simulink model "CM640A_MotAg1Meas"  (R2013b)
settings: Solver=FixedStepDiscrete  SolverMode=SingleTasking  StartTime=0.0  StopTime=1  FixedStep=0.0000625  RelTol=1e-3
undefined symbols (not defined in the file): ARCHGLBPRM_2PI_ULS_F32, COEFFTBLELMSIZE_CNT_U08, COEFFTBLSIZE_CNT_U08, CORRNTBLAGSTEPSIZE_MATRAD_F32, CORRNTBLSIDXOFFS_CNT_U16, CORRNTBLSIZE_CNT_U16, CORRNTBLSIZEMASK_CNT_U08, MOTAG1OFFS_MOTREV_U0P16, MotAg1PrtclFlt, MOTAG1PRTCLFLTFAILSTEP_CNT_U16, MOTAG1PRTCLFLTPASSSTEP_CNT_U16, MOTAGDELTAPERCORRNPT_CNT_U16, MOTAGIDXMASK_CNT_U16, MotCtrlMotAg1ErrReg, NtcSts1, sigbuilder_block, SNSRAGMASK_CNT_U32, SNSRERRMASK_CNT_U32, SNSRERRNTCMASK_CNT_U08, SNSRVLTGFLTMASK_CNT_U32, SPIPARMASK_CNT_U32
libraries: simulink x28, FloatToFixd x1, NxtrMax x1, NxtrLim x1
(part 1 of 4)
settings Model: RequirementInfo="{}  %GIDa_ca294f38_ed7c_4fb9_8c54_f4d56271bfc7"  ModifiedHistory=Rev 008: Updated model to Matlab 2013B, added comments to show requirement linkage  Creator=nz3zln  LastModifiedBy=FZG88Y
settings SolverCC: AutoInsertRateTranBlk=on  InsertRTBMode=Always
settings DataIOCC: LimitDataPoints=off  SaveFormat=Structure  ReturnWorkspaceOutputs=on
settings OptimizationCC: BlockReduction=off  InlineParams=on  ZeroExternalMemoryAtStartup=off  ZeroInternalMemoryAtStartup=off  OptimizeModelRefInitCode=on  LifeSpan=1
settings DebuggingCC: SignalInfNanChecking=error  SignalRangeChecking=warning  UnderspecifiedInitializationDetection=Simplified  SolverPrmCheckMsg=error  InheritedTsInSrcMsg=error  DiscreteInheritContinuousMsg=error  SingleTaskRateTransMsg=error  TasksWithSamePriorityMsg=error  SigSpecEnsureSampleTimeMsg=error  CheckMatrixSingularityMsg=error  ParameterUnderflowMsg=error  ParameterPrecisionLossMsg=error  ParameterTunabilityLossMsg=error  FixptConstUnderflowMsg=warning  FixptConstOverflowMsg=warning  VectorMatrixConversionMsg=error  SignalLabelMismatchMsg=error  UnconnectedInputMsg=error  UnconnectedOutputMsg=error  UnconnectedLineMsg=error  SFcnCompatibilityMsg=error  UniqueDataStoreMsg=warning  BusObjectLabelMismatch=error  RootOutportRequireBusObject=error  AssertControl=DisableAll  ModelReferenceIOMsg=error  ModelReferenceVersionMismatchMessage=warning  ModelReferenceIOMismatchMessage=error  ModelReferenceCSMismatchMessage=warning  ModelReferenceDataLoggingMessage=error  StateNameClashWarn=warning  StrictBusMsg=ErrorOnBusTreatedAsVector  NonBusSignalsTreatedAsBus=error  SFUnexpectedBacktrackingDiag=error  SFInvalidInputDataAccessInChartInitDiag=error  SFNoUnconditionalDefaultTransitionDiag=error  SFTransitionOutsideNaturalParentDiag=error  SFUnconditionalTransitionShadowingDiag=error  SFUndirectedBroadcastEventsDiag=error
settings ModelReferenceCC: ModelReferenceNumInstancesAllowed=Single
settings RTWCC: SystemTargetFile=autosar.tlc  GenCodeOnly=on  TemplateMakefile=ert_default_tmf  Description=AUTOSAR  GenerateReport=on  ProcessScript=autosar_make_rtw_hook  LaunchReport=on
settings CodeAppCC: GenerateComments=off  IgnoreCustomStorageClasses=off  CustomSymbolStrType=$N$R$M  CustomSymbolStrBlkIO=$N$M  SimulinkBlockComments=off
settings STFCustomTargetCC: ParMdlRefBuildCompliant=on  CompOptLevelCompliant=on  IncludeMdlTerminateFcn=off  CombineOutputUpdateFcns=on  SuppressErrorStatus=on  ERTFirstTimeCompliant=on  ERTCustomFileBanners=on  SupportNonFinite=off  SupportComplex=off  SupportContinuousTime=off  SupportNonInlinedSFcns=off  MATLABClassNameForMDSCustomization=Simulink.SoftwareTarget.ERTCustomization  AutosarCompliant=on  GRTInterface=off  SystemTargetFile=autosar.tlc
settings ERTTargetCC: CodeReplacementLibrary=ANSI_C  ConcurrentExecutionCompliant=off  IncludeMdlTerminateFcn=off  SuppressErrorStatus=on  SupportNonFinite=off  SupportComplex=off  ModelStepFunctionPrototypeControlCompliant=off  CPPClassGenCompliant=off  AutosarCompliant=on  InlinedParameterPlacement=NonHierarchical  ERTCustomFileTemplate=example_file_process.tlc  EnableUserReplacementTypes=on

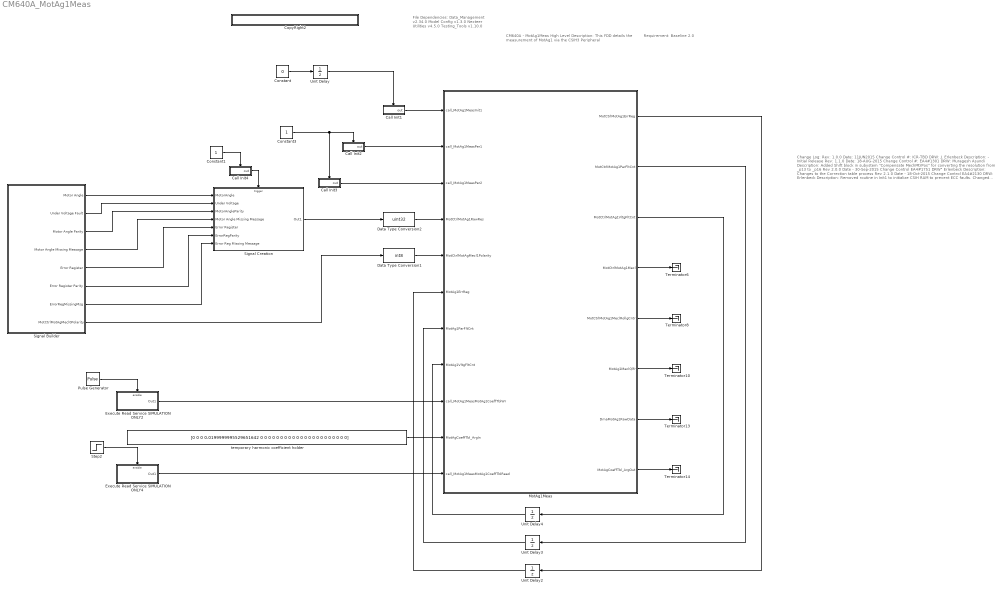
== system CM640A_MotAg1Meas ==
  note: CM640A - MotAg1Meas
      |
      | High Level Description:
      | This FDD details the measurement of MotAg1 via the CSIH3 Peripheral
  note: Change Log:
      |
      | Rev: 1.0.0
      | Date: 11JUN2015
      | Change Control #: ICR-TBD
      | DRW: J. Erlenbeck
      | Description:
      | - Initial Release
      |
      | Rev: 1.1.0
      | Date: 18-AUG-2015
      | Change Control #: EA4#1301
      | DRW: Muragesh Asundi
      | Description: Added Shift block in subystem "Compensate MechMtrPos" for converting the resolution from _p13 to _p16
      |
      | Rev 2.0.0
      | Date - 30-Sep-2015
      | Change Control EA4#1751
      | DRW" Erlenbeck
      | Description: Changes to the Correction table process
      |
      | Rev 2.1.0
      | Date -  18-Oct-2015
      | Change Control EA4#2130
      | DRW: Erlenbeck
      | Description: Removed routine in Init1 to initialize CSIH RAM to prevent ECC faults.  Changed some
      | typecasting in init function that prevented the function from running when NxtrMBDConfig.mat was run.
      | Replaced input signal creation from external file to one with signal builder.
      |
      | Rev 2.4.0
      | Date -  17-Dec-2015
      | Change Control EA4#3209
      | DRW: Erlenbeck
      | Description: Removed read reset pointer
      |
      | Rev 2.5.0
      | Date -  08-Mar-2016
      | Change Control EA4#3999, EA4#4646
      | DRW: Praveen(KPIT)
      | Description: -
      | - M File change so that NVM MotAg1CoeffTbl.EngInit = []. Accordingly model updated to allign to this.
      | - As per anomaly CR EA4#3631, updated the Variable MotCtrlMotAg1VltgFltCnt.WrittenIn field as MotAg1MeasPer1 in the .m file.
      | - The maximum and minimum specified in the Data Type conversion block are removed and highlighted in the Model.
      | - Server runnable name changed from MotAg0MeasMotAg1CoeffTblRead to MotAg1MeasMotAg1CoeffTblRead.
  note: File Dependencies:
      | Data_Management v2.34.0
      | Model Config v1.3.0
      | Nexteer Utilities v4.5.0
      | Testing_Tools v1.10.0
  note: Requirement: Baseline 2.0
  Call Init1 : Subsystem  TreatAsAtomicUnit=on
  Call Init2 : Subsystem  TreatAsAtomicUnit=on
  Call Init3 : Subsystem  TreatAsAtomicUnit=on
  Call Init4 : Subsystem  TreatAsAtomicUnit=on
  Constant : Constant  Value=0  OutDataTypeStr=uint8
  Constant1 : Constant  OutDataTypeStr=int8
  Constant3 : Constant  OutDataTypeStr=int8
  CopyRight2 : Subsystem  Description=|  mask(Copyright Information){none=on}
      | Copyright info block.                                               
      |                                                                     
      | Place copyright information at the top of every subsystem in design.
      mask prompts: none "No parameters"
      mask help: Place copyright information at the top of every subsystem in design.
      mask Display:
      | NxtrConf = 'Nexteer Confidential';
      | 
      | sys = bdroot; %handle for the current model ("system")
      | first = get_param(sys,'Created');
      | first = first(end-3:end);  %year is last four digits
      | 
      | last = get_param(sys,'LastModifiedDate');
      | if isempty(last)
      |     last = datestr(now,'yyyy');
      | else
      |     last = last(end-3:end);
      | end
      | 
      | if strcmp(first,last)
      |     fprintf('%s -- Copyright %s Nexteer',NxtrConf,first)
      | else
      |     fprintf('%s -- %s%s- %s Nexteer',NxtrConf,char(169),first,last)
      | end
  Data Type Conversion1 : DataTypeConversion  OutDataTypeStr=int8
  Data Type Conversion2 : DataTypeConversion  OutDataTypeStr=uint32
  Execute Read Service SIMULATION ONLY2 : Subsystem  TreatAsAtomicUnit=on
  Execute Read Service SIMULATION ONLY4 : Subsystem  TreatAsAtomicUnit=on
  MotAg1Meas : Subsystem
  Pulse Generator : DiscretePulseGenerator  PulseType=Time based  Period=1  PhaseDelay=0.6
  Signal Builder : Subsystem  Tag=STV Subsys  LoadFcn=sigbuilder_block('load');  StartFcn=sigbuilder_block('start');  StopFcn=sigbuilder_block('stop');  ClipboardFcn=sigbuilder_block('clipboard');  mask(Sigbuilder block){}
      mask help: Simulink:masks:SigbuilderBlock_MD
      mask init:
      | if ~strcmp(get_param(bdroot(gcbh),'SimulationStatus'),'stopped') tuvar = sigbuilder_block('maskInit'); end
      settings: CopyFcn=sigbuilder_block('copy');  DeleteFcn=sigbuilder_block('delete');  ModelCloseFcn=sigbuilder_block('modelClose');  PreSaveFcn=sigbuilder_block('preSave');  PauseFcn=sigbuilder_block('pause');  ContinueFcn=sigbuilder_block('continue');  NameChangeFcn=sigbuilder_block('namechange');  OpenFcn=sigbuilder_block('open',[306 215.379 548.69 396.621 ]);  CloseFcn=sigbuilder_block('close');
      mask Display: plot(0, 0, 100, 100,[2, 2, 32, 32, 2], [68, 8, 8, 68, 68],[32, 2], [38, 38], [32, 19, 2],[53, 60, 44], [32, 17, 17, 2],[16, 16, 31, 31]);txt = getActiveGroup(gcbh);text(2, 100, txt,'verticalAlignment', 'top');
  Signal Creation : Subsystem
  Step2 : Step  Time=0.8  SampleTime=0
  Terminator{6,8,10,13..14} (5 alike) : Terminator
  Unit Delay : UnitDelay  InitialCondition=1  SampleTime=-1
  Unit Delay2 : UnitDelay  SampleTime=-1
  Unit Delay3 : UnitDelay  SampleTime=-1
  Unit Delay4 : UnitDelay  SampleTime=-1
  temporary harmonic coefficient holder : Constant  Value=[0 0 0 0.0199999995529651642 0 0 0 0 0 0 0 0 0 0 0 0 0 0 0 0 0 0 0 0 0 0]  OutDataTypeStr=single
  wires:
  Constant/1 -> Unit Delay/1
  Unit Delay/1 -> Call Init1/Enable
  Constant3/1 -> Call Init2/Enable, Call Init3/Enable
  Call Init1/1(out) -> MotAg1Meas/1(call_MotAg1MeasInit1)
  Call Init2/1(out) -> MotAg1Meas/2(call_MotAg1MeasPer1)
  Call Init3/1(out) -> MotAg1Meas/3(call_MotAg1MeasPer2)
  MotAg1Meas/4(MotCtrlMotAg1Mecl) -> Terminator6/1
  MotAg1Meas/5(MotCtrlMotAg1MeclRollgCntr) -> Terminator8/1
  MotAg1Meas/6(MotAg1MeclQlfr) -> Terminator10/1
  MotAg1Meas/7(DmaMotAg1RawData) -> Terminator13/1
  Pulse Generator/1 -> Execute Read Service SIMULATION ONLY2/Enable
  Step2/1 -> Execute Read Service SIMULATION ONLY4/Enable
  MotAg1Meas/1(MotCtrlMotAg1ErrReg) -> Unit Delay2/1
  Unit Delay2/1 -> MotAg1Meas/6(MotAg1ErrReg)
  MotAg1Meas/2(MotCtrlMotAg1ParFltCnt) -> Unit Delay3/1
  Unit Delay3/1 -> MotAg1Meas/7(MotAg1ParFltCnt)
  MotAg1Meas/3(MotCtrlMotAg1VltgFltCnt) -> Unit Delay4/1
  Unit Delay4/1 -> MotAg1Meas/8(MotAg1VltgFltCnt)
  MotAg1Meas/8(MotAgCoeffTbl_ArgOut) -> Terminator14/1
  Execute Read Service SIMULATION ONLY2/1(Out1) -> MotAg1Meas/9(call_MotAg1MeasMotAg1CoeffTblWr)
  Execute Read Service SIMULATION ONLY4/1(Out1) -> MotAg1Meas/11(call_MotAg1MeasMotAg1CoeffTblRead)
  temporary harmonic coefficient holder/1 -> MotAg1Meas/10(MotAgCoeffTbl_ArgIn)
  Signal Creation/1(Out1) -> Data Type Conversion2/1
  Constant1/1 -> Call Init4/Enable
  Call Init4/1(out) -> Signal Creation/Trigger
  Signal Builder/1(Motor Angle) -> Signal Creation/1(MotorAngle)
  Signal Builder/2(Under Voltage Fault) -> Signal Creation/2(Under Voltage)
  Signal Builder/3(Motor Angle Parity) -> Signal Creation/3(MotorAngleParity)
  Signal Builder/5(Error Register) -> Signal Creation/5(Error Register)
  Signal Builder/6(Error Register Parity) -> Signal Creation/6(ErrorRegParity)
  Signal Builder/8(MotCtrlMotAgMecl0Polarity) -> Data Type Conversion1/1
  Signal Builder/4(Motor Angle Missing Message) -> Signal Creation/4(Motor Angle Missing Message)
  Signal Builder/7(ErrorRegMissingMsg) -> Signal Creation/7(Error Reg Missing Message)
  Data Type Conversion2/1 -> MotAg1Meas/4(MotCtrlMotAg1RawRes)
  Data Type Conversion1/1 -> MotAg1Meas/5(MotCtrlMotAgMecl1Polarity)

== system CM640A_MotAg1Meas/Call Init1 ==
  Enable : EnablePort
  Function Call Trigger : simulink/Ports & Subsystems/Function-Call Generator  RequirementInfo={} %GIDa_ff755a2e_49d1_45f7_8591_3ce0ef475338  sample_time=0.002  numberOfIterations=1
  out : Outport
  wires:
  Function Call Trigger/1 -> out/1

== system CM640A_MotAg1Meas/Call Init2 ==
  Enable : EnablePort
  Function Call Trigger : simulink/Ports & Subsystems/Function-Call Generator  RequirementInfo={} %GIDa_6dd05ab1_f91b_4d7a_a0ec_1170d213fa7b  sample_time=0.0005  numberOfIterations=1
  out : Outport
  wires:
  Function Call Trigger/1 -> out/1

== system CM640A_MotAg1Meas/Call Init3 ==
  Enable : EnablePort
  Function Call Trigger : simulink/Ports & Subsystems/Function-Call Generator  RequirementInfo={} %GIDa_9bd65ccd_39f3_4e48_9d09_4984d13bbcbb  sample_time=0.002  numberOfIterations=1
  out : Outport
  wires:
  Function Call Trigger/1 -> out/1

== system CM640A_MotAg1Meas/Call Init4 ==
  Enable : EnablePort
  Function Call Trigger : simulink/Ports & Subsystems/Function-Call Generator  RequirementInfo={} %GIDa_6dd05ab1_f91b_4d7a_a0ec_1170d213fa7b  sample_time=0.0005  numberOfIterations=1
  out : Outport
  wires:
  Function Call Trigger/1 -> out/1

== system CM640A_MotAg1Meas/CopyRight2 ==

== system CM640A_MotAg1Meas/Execute Read Service SIMULATION ONLY2 ==
  Enable : EnablePort
  Function-Call Generator1 : simulink/Ports & Subsystems/Function-Call Generator  sample_time=0.0000625  numberOfIterations=1
  Out1 : Outport
  wires:
  Function-Call Generator1/1 -> Out1/1

== system CM640A_MotAg1Meas/Execute Read Service SIMULATION ONLY4 ==
  Enable : EnablePort
  Function-Call Generator1 : simulink/Ports & Subsystems/Function-Call Generator  sample_time=0.0000625  numberOfIterations=1
  Out1 : Outport
  wires:
  Function-Call Generator1/1 -> Out1/1

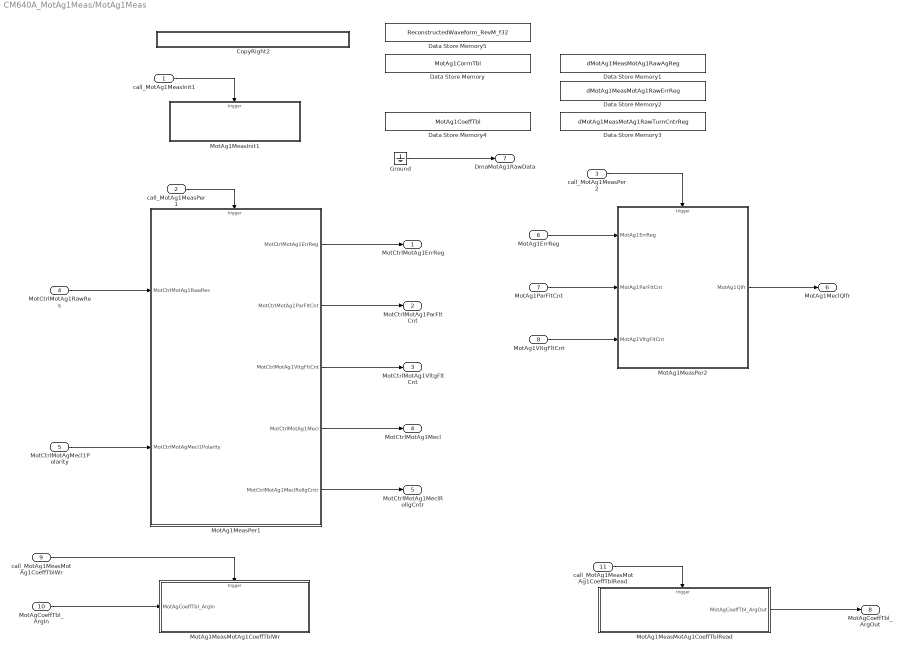
== system CM640A_MotAg1Meas/MotAg1Meas ==
  call_MotAg1MeasInit1 : Inport  RequirementInfo={} %GIDa_18b4b7a7_d8ff_42fd_afd9_8fbc558fb7ae
  call_MotAg1MeasPer1 : Inport  RequirementInfo={} %GIDa_8c56c68f_1996_47ee_bda4_35b4dc112bcf  Port=2
  call_MotAg1MeasPer2 : Inport  RequirementInfo={} %GIDa_7b28921c_189e_46dc_b03b_f7509365a7f9  Port=3
  MotCtrlMotAg1RawRes : Inport  RequirementInfo={} %GIDa_768985a4_e900_425c_ae1d_47338650e664  Port=4
  MotCtrlMotAgMecl1Polarity : Inport  RequirementInfo={} %GIDa_8ed9d5d5_f39e_4ce8_8e17_7324d3fb8e4d  Port=5  OutDataTypeStr=int8
  MotAg1ErrReg : Inport  Port=6
  MotAg1ParFltCnt : Inport  Port=7
  MotAg1VltgFltCnt : Inport  Port=8
  call_MotAg1MeasMotAg1CoeffTblWr : Inport  Port=9
  MotAgCoeffTbl_ArgIn : Inport  Port=10
  call_MotAg1MeasMotAg1CoeffTblRead : Inport  Port=11
  CopyRight2 : Subsystem  Description=|  mask(Copyright Information){none=on}
      | Copyright info block.                                               
      |                                                                     
      | Place copyright information at the top of every subsystem in design.
      mask prompts: none "No parameters"
      mask help: Place copyright information at the top of every subsystem in design.
      mask Display:
      | NxtrConf = 'Nexteer Confidential';
      | 
      | sys = bdroot; %handle for the current model ("system")
      | first = get_param(sys,'Created');
      | first = first(end-3:end);  %year is last four digits
      | 
      | last = get_param(sys,'LastModifiedDate');
      | if isempty(last)
      |     last = datestr(now,'yyyy');
      | else
      |     last = last(end-3:end);
      | end
      | 
      | if strcmp(first,last)
      |     fprintf('%s -- Copyright %s Nexteer',NxtrConf,first)
      | else
      |     fprintf('%s -- %s%s- %s Nexteer',NxtrConf,char(169),first,last)
      | end
  Data Store Memory : DataStoreMemory  DataStoreName=MotAg1CorrnTbl  InitialValue=[]  StateMustResolveToSignalObject=on
  Data Store Memory1 : DataStoreMemory  DataStoreName=dMotAg1MeasMotAg1RawAgReg  OutDataTypeStr=uint32  StateMustResolveToSignalObject=on
  Data Store Memory2 : DataStoreMemory  DataStoreName=dMotAg1MeasMotAg1RawErrReg  OutDataTypeStr=uint32  StateMustResolveToSignalObject=on
  Data Store Memory3 : DataStoreMemory  DataStoreName=dMotAg1MeasMotAg1RawTurnCntrReg  OutDataTypeStr=uint32  StateMustResolveToSignalObject=on
  Data Store Memory4 : DataStoreMemory  DataStoreName=MotAg1CoeffTbl  InitialValue=[]  StateMustResolveToSignalObject=on
  Data Store Memory5 : DataStoreMemory  DataStoreName=ReconstructedWaveform_RevM_f32  InitialValue=zeros(128,1)  OutDataTypeStr=single
  Ground : Ground
  MotAg1MeasInit1 : Subsystem
  MotAg1MeasMotAg1CoeffTblRead : Subsystem  RequirementInfo="{'linktype_rmi_doors' '0000cf48 (/ESG Group/FDD Module Requirements/EA4 Specific/CM640A_MotAg1Meas)' '#CM640A_116' 'true' 'REQ:  CM640A_116' '' } %GIDa_cbbcdd8d_f009_454c_a06b_3b2ba8e819d4"
  MotAg1MeasMotAg1CoeffTblWr : Subsystem  RequirementInfo="{'linktype_rmi_doors' '0000cf48 (/ESG Group/FDD Module Requirements/EA4 Specific/CM640A_MotAg1Meas)' '#CM640A_115' 'true' 'REQ:  CM640A_115' '' } %GIDa_0a2db888_59fe_4955_b15e_b7f61818f82e"
  MotAg1MeasPer1 : Subsystem  TreatAsAtomicUnit=on
  MotAg1MeasPer2 : Subsystem  TreatAsAtomicUnit=on
  MotCtrlMotAg1ErrReg : Outport
  MotCtrlMotAg1ParFltCnt : Outport  Port=2
  MotCtrlMotAg1VltgFltCnt : Outport  Port=3
  MotCtrlMotAg1Mecl : Outport  RequirementInfo={} %GIDa_a40ef296_4e6e_4397_997e_05fcb9e70ed5  Port=4
  MotCtrlMotAg1MeclRollgCntr : Outport  Port=5
  MotAg1MeclQlfr : Outport  RequirementInfo={} %GIDa_eb095ceb_60c6_4658_947c_a9047682a36a  Port=6
  DmaMotAg1RawData : Outport  Port=7
  MotAgCoeffTbl_ArgOut : Outport  Port=8
  wires:
  MotCtrlMotAgMecl1Polarity/1 -> MotAg1MeasPer1/2(MotCtrlMotAgMecl1Polarity)
  call_MotAg1MeasInit1/1 -> MotAg1MeasInit1/Trigger
  call_MotAg1MeasPer1/1 -> MotAg1MeasPer1/Trigger
  MotCtrlMotAg1RawRes/1 -> MotAg1MeasPer1/1(MotCtrlMotAg1RawRes)
  MotAg1MeasPer1/1(MotCtrlMotAg1ErrReg) -> MotCtrlMotAg1ErrReg/1
  MotAg1MeasPer1/3(MotCtrlMotAg1VltgFltCnt) -> MotCtrlMotAg1VltgFltCnt/1
  MotAg1MeasPer1/2(MotCtrlMotAg1ParFltCnt) -> MotCtrlMotAg1ParFltCnt/1
  MotAg1MeasPer1/4(MotCtrlMotAg1Mecl) -> MotCtrlMotAg1Mecl/1
  MotAg1MeasPer1/5(MotCtrlMotAg1MeclRollgCntr) -> MotCtrlMotAg1MeclRollgCntr/1
  call_MotAg1MeasPer2/1 -> MotAg1MeasPer2/Trigger
  MotAg1ErrReg/1 -> MotAg1MeasPer2/1(MotAg1ErrReg)
  MotAg1ParFltCnt/1 -> MotAg1MeasPer2/2(MotAg1ParFltCnt)
  MotAg1VltgFltCnt/1 -> MotAg1MeasPer2/3(MotAg1VltgFltCnt)
  MotAg1MeasPer2/1(MotAg1Qlfr) -> MotAg1MeclQlfr/1
  Ground/1 -> DmaMotAg1RawData/1
  call_MotAg1MeasMotAg1CoeffTblWr/1 -> MotAg1MeasMotAg1CoeffTblWr/Trigger
  MotAgCoeffTbl_ArgIn/1 -> MotAg1MeasMotAg1CoeffTblWr/1(MotAgCoeffTbl_ArgIn)
  call_MotAg1MeasMotAg1CoeffTblRead/1 -> MotAg1MeasMotAg1CoeffTblRead/Trigger
  MotAg1MeasMotAg1CoeffTblRead/1(MotAgCoeffTbl_ArgOut) -> MotAgCoeffTbl_ArgOut/1

== system CM640A_MotAg1Meas/Signal Builder ==
  Demux : Demux  Tag=STV Demux  Outputs=8
  FromWs : FromWorkspace  Tag=STV FromWs  VariableName=tuvar  SampleTime=0
      SigBuilderData=|
      | common.afterFinalStr = 'Extrapolate'
      | common.sampleTime = 0
      | dataSet.timeRange = [0 2]
      | dataSet.name = 'Group 1'
      | sbobj.Groups.Name = 'Group 1'
      | sbobj.Groups.Signals(1).Name = 'Motor Angle'
      | sbobj.Groups.Signals(1).XData = [0 1 2]
      | sbobj.Groups.Signals(1).YData = [0 1500 -900]
      | sbobj.Groups.Signals(2).Name = 'Under Voltage Fault'
      | sbobj.Groups.Signals(2).XData = [0 0.288 0.288 0.326 0.326 2]
      | sbobj.Groups.Signals(2).YData = [0 0 1 1 0 0]
      | sbobj.Groups.Signals(3).Name = 'Motor Angle Parity'
      | sbobj.Groups.Signals(3).XData = [0 0.201 0.201 0.21 0.21 2]
      | sbobj.Groups.Signals(3).YData = [0 0 1 1 0 0]
      | sbobj.Groups.Signals(4).Name = 'Motor Angle Missing Message'
      | sbobj.Groups.Signals(4).XData = [0 0.534 0.534 0.544 0.544 2]
      | sbobj.Groups.Signals(4).YData = [0 0 1 1 0 0]
      | sbobj.Groups.Signals(5).Name = 'Error Register'
      | sbobj.Groups.Signals(5).XData = [0 0.864 0.864 0.898 0.898 0.962 0.962 1.056 1.056 1.144 1.144 1.2 1.2 1.264 1.264 2]
      | sbobj.Groups.Signals(5).YData = [0 0 1 1 2 2 4 4 0 0 8 8 6 6 0 0]
      | sbobj.Groups.Signals(6).Name = 'Error Register Parity'
      | sbobj.Groups.Signals(6).XData = [0 2]
      | sbobj.Groups.Signals(6).YData = [0 0]
      | sbobj.Groups.Signals(7).Name = 'ErrorRegMissingMsg'
      | sbobj.Groups.Signals(7).XData = [0 1.608 1.608 1.632 1.632 2]
      | sbobj.Groups.Signals(7).YData = [0 0 1 1 0 0]
      | sbobj.Groups.Signals(8).Name = 'MotCtrlMotAgMecl0Polarity'
      | sbobj.Groups.Signals(8).XData = [0 1.792 1.792 2]
      | sbobj.Groups.Signals(8).YData = [1 1 -1 -1]
      | sbobj.Groups.TimeRange = [0 2]
  Motor Angle : Outport  Tag=STV Outport
  Under Voltage Fault : Outport  Tag=STV Outport  Port=2
  Motor Angle Parity : Outport  Tag=STV Outport  Port=3
  Motor Angle Missing Message : Outport  Tag=STV Outport  Port=4
  Error Register : Outport  Tag=STV Outport  Port=5
  Error Register Parity : Outport  Tag=STV Outport  Port=6
  ErrorRegMissingMsg : Outport  Tag=STV Outport  Port=7
  MotCtrlMotAgMecl0Polarity : Outport  Tag=STV Outport  Port=8
  wires:
  FromWs/1 -> Demux/1
  Demux/1 -> Motor Angle/1
  Demux/2 -> Under Voltage Fault/1
  Demux/3 -> Motor Angle Parity/1
  Demux/4 -> Motor Angle Missing Message/1
  Demux/5 -> Error Register/1
  Demux/6 -> Error Register Parity/1
  Demux/7 -> ErrorRegMissingMsg/1
  Demux/8 -> MotCtrlMotAgMecl0Polarity/1

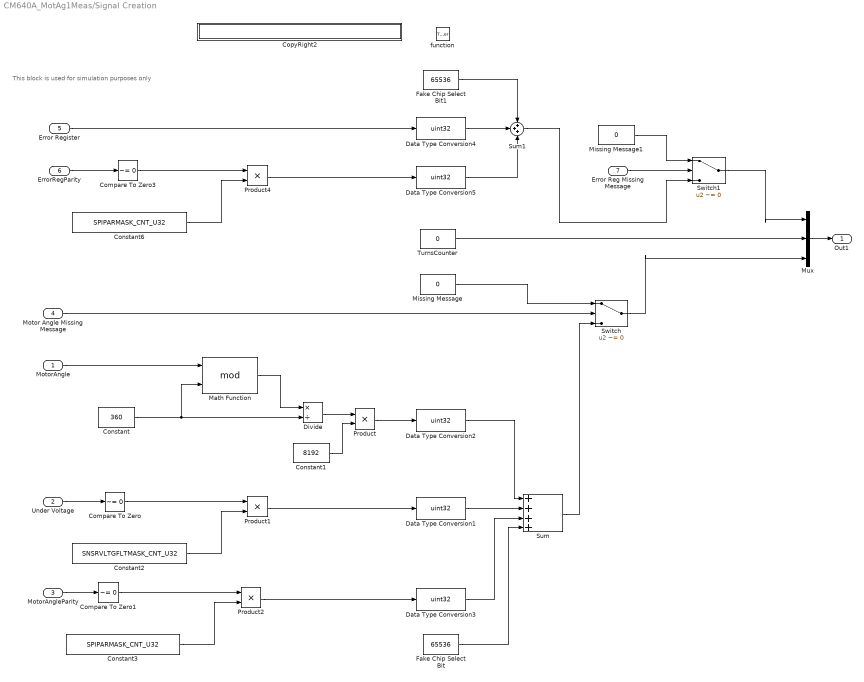
== system CM640A_MotAg1Meas/Signal Creation ==
  note: This block is used for simulation purposes only
  MotorAngle : Inport  RequirementInfo={} %GIDa_5b9207d5_047a_4d13_ad58_24937db38f49
  Under Voltage : Inport  RequirementInfo={} %GIDa_49b5407c_b803_41d3_a0e6_5a24965301ee  Port=2
  MotorAngleParity : Inport  RequirementInfo={} %GIDa_e27ee528_5af8_4fa8_b3a6_ac23e448c106  Port=3
  Motor Angle Missing Message : Inport  RequirementInfo={} %GIDa_65758099_f818_4bb9_9018_519c50253ef5  Port=4
  Error Register : Inport  RequirementInfo={} %GIDa_a9b16e92_8e1c_4949_a94d_59951fb47bd4  Port=5
  ErrorRegParity : Inport  RequirementInfo={} %GIDa_65ea76fc_4001_4f2e_a8c7_2b1e4b6c204c  Port=6
  Error Reg Missing Message : Inport  RequirementInfo={} %GIDa_41a49761_6592_496d_8eb4_6dd2a2fb863d  Port=7
  function : TriggerPort  TriggerType=function-call
  Compare To Zero : simulink/Logic and Bit Operations/Compare To Zero  relop=~=  OutDataTypeStr=uint8
  Compare To Zero1 : simulink/Logic and Bit Operations/Compare To Zero  relop=~=  OutDataTypeStr=uint8
  Compare To Zero3 : simulink/Logic and Bit Operations/Compare To Zero  relop=~=  OutDataTypeStr=uint8
  Constant : Constant  Value=360
  Constant1 : Constant  Value=8192
  Constant2 : Constant  Value=SNSRVLTGFLTMASK_CNT_U32
  Constant3 : Constant  Value=SPIPARMASK_CNT_U32
  Constant6 : Constant  Value=SPIPARMASK_CNT_U32
  CopyRight2 : Subsystem  Description=|  mask(Copyright Information){none=on}
      | Copyright info block.                                               
      |                                                                     
      | Place copyright information at the top of every subsystem in design.
      mask prompts: none "No parameters"
      mask help: Place copyright information at the top of every subsystem in design.
      mask Display:
      | NxtrConf = 'Nexteer Confidential';
      | 
      | sys = bdroot; %handle for the current model ("system")
      | first = get_param(sys,'Created');
      | first = first(end-3:end);  %year is last four digits
      | 
      | last = get_param(sys,'LastModifiedDate');
      | if isempty(last)
      |     last = datestr(now,'yyyy');
      | else
      |     last = last(end-3:end);
      | end
      | 
      | if strcmp(first,last)
      |     fprintf('%s -- Copyright %s Nexteer',NxtrConf,first)
      | else
      |     fprintf('%s -- %s%s- %s Nexteer',NxtrConf,char(169),first,last)
      | end
  Data Type Conversion{1..5} (5 alike) : DataTypeConversion  OutDataTypeStr=uint32
  Divide : Product  Inputs=*/
  Fake Chip Select Bit : Constant  Value=65536  OutDataTypeStr=uint32
  Fake Chip Select Bit1 : Constant  Value=65536  OutDataTypeStr=uint32
  Math Function : Math  Operator=mod  SaturateOnIntegerOverflow=on
  Missing Message : Constant  Value=0  OutDataTypeStr=uint32
  Missing Message1 : Constant  Value=0  OutDataTypeStr=uint32
  Mux : Mux  Inputs=3
  Product{,1..2,4} (4 alike) : Product
  Sum : Sum  Inputs=++++
  Sum1 : Sum  Inputs=+++
  Switch : Switch  Criteria=u2 ~= 0
  Switch1 : Switch  Criteria=u2 ~= 0
  TurnsCounter : Constant  Value=0  OutDataTypeStr=uint32
  Out1 : Outport
  wires:
  MotorAngle/1 -> Math Function/1
  Constant/1 -> Math Function/2, Divide/2
  Math Function/1 -> Divide/1
  Divide/1 -> Product/1
  Constant1/1 -> Product/2
  Product/1 -> Data Type Conversion2/1
  Mux/1 -> Out1/1
  Under Voltage/1 -> Compare To Zero/1
  Compare To Zero/1 -> Product1/1
  Constant2/1 -> Product1/2
  MotorAngleParity/1 -> Compare To Zero1/1
  Compare To Zero1/1 -> Product2/1
  Constant3/1 -> Product2/2
  Data Type Conversion2/1 -> Sum/1
  Product1/1 -> Data Type Conversion1/1
  Product2/1 -> Data Type Conversion3/1
  Data Type Conversion1/1 -> Sum/2
  Data Type Conversion3/1 -> Sum/3
  TurnsCounter/1 -> Mux/2
  ErrorRegParity/1 -> Compare To Zero3/1
  Compare To Zero3/1 -> Product4/1
  Constant6/1 -> Product4/2
  Product4/1 -> Data Type Conversion5/1
  Sum1/1 -> Switch1/3
  Error Register/1 -> Data Type Conversion4/1
  Fake Chip Select Bit/1 -> Sum/4
  Motor Angle Missing Message/1 -> Switch/2
  Missing Message/1 -> Switch/1
  Sum/1 -> Switch/3
  Switch/1 -> Mux/3
  Missing Message1/1 -> Switch1/1
  Error Reg Missing Message/1 -> Switch1/2
  Switch1/1 -> Mux/1
  Fake Chip Select Bit1/1 -> Sum1/1
  Data Type Conversion4/1 -> Sum1/2
  Data Type Conversion5/1 -> Sum1/3

== system CM640A_MotAg1Meas/MotAg1Meas/CopyRight2 ==

== system CM640A_MotAg1Meas/MotAg1Meas/MotAg1MeasInit1 ==
  function : TriggerPort  TriggerType=function-call
  Compute Correction Table : Subsystem  Priority=30  TreatAsAtomicUnit=on
      settings: AttributesFormatString=|
      | Priority:
      | %<Priority>
  CopyRight2 : Subsystem  Description=|  mask(Copyright Information){none=on}
      | Copyright info block.                                               
      |                                                                     
      | Place copyright information at the top of every subsystem in design.
      mask prompts: none "No parameters"
      mask help: Place copyright information at the top of every subsystem in design.
      mask Display:
      | NxtrConf = 'Nexteer Confidential';
      | 
      | sys = bdroot; %handle for the current model ("system")
      | first = get_param(sys,'Created');
      | first = first(end-3:end);  %year is last four digits
      | 
      | last = get_param(sys,'LastModifiedDate');
      | if isempty(last)
      |     last = datestr(now,'yyyy');
      | else
      |     last = last(end-3:end);
      | end
      | 
      | if strcmp(first,last)
      |     fprintf('%s -- Copyright %s Nexteer',NxtrConf,first)
      | else
      |     fprintf('%s -- %s%s- %s Nexteer',NxtrConf,char(169),first,last)
      | end
  Initialize CSIH RAM1 : Subsystem  Priority=20  TreatAsAtomicUnit=on
      settings: AttributesFormatString=|
      | Priority:
      | %<Priority>

== system CM640A_MotAg1Meas/MotAg1Meas/MotAg1MeasMotAg1CoeffTblRead ==
  Trigger : TriggerPort  TriggerType=function-call  PortDimensions=1
  Copyright1 : Subsystem  Description=|  mask(Copyright Information){none=on}
      | Copyright info block.                                               
      |                                                                     
      | Place copyright information at the top of every subsystem in design.
      mask prompts: none "No parameters"
      mask help: Place copyright information at the top of every subsystem in design.
      mask Display:
      | NxtrConf = 'Nexteer Confidential';
      | 
      | sys = bdroot; %handle for the current model ("system")
      | first = get_param(sys,'Created');
      | if(isempty(first))
      |     first = datestr(now,'yyyy');
      | else
      |     first = first(end-3:end);  %year is last four digits
      | end
      | 
      | last = get_param(sys,'LastModifiedDate');
      | if isempty(last)
      |     last = datestr(now,'yyyy');
      | else
      |     last = last(end-3:end);
      | end
      | 
      | if strcmp(first,last)
      |     fprintf('%s\nCopyright  %s Nexteer',NxtrConf,first);
      | else
      |     fprintf('%s\n%s%s-%s Nexteer',NxtrConf,char(169),first,last);
      | end
  Data Store Read : DataStoreRead  DataStoreName=MotAg1CoeffTbl
  MotAgCoeffTbl_ArgOut : Outport
  wires:
  Data Store Read/1 -> MotAgCoeffTbl_ArgOut/1

== system CM640A_MotAg1Meas/MotAg1Meas/MotAg1MeasMotAg1CoeffTblWr ==
  MotAgCoeffTbl_ArgIn : Inport
  Trigger : TriggerPort  TriggerType=function-call  PortDimensions=1
  Block Changed = True : Constant  OutDataTypeStr=boolean
  Copyright1 : Subsystem  Description=|  mask(Copyright Information){none=on}
      | Copyright info block.                                               
      |                                                                     
      | Place copyright information at the top of every subsystem in design.
      mask prompts: none "No parameters"
      mask help: Place copyright information at the top of every subsystem in design.
      mask Display:
      | NxtrConf = 'Nexteer Confidential';
      | 
      | sys = bdroot; %handle for the current model ("system")
      | first = get_param(sys,'Created');
      | if(isempty(first))
      |     first = datestr(now,'yyyy');
      | else
      |     first = first(end-3:end);  %year is last four digits
      | end
      | 
      | last = get_param(sys,'LastModifiedDate');
      | if isempty(last)
      |     last = datestr(now,'yyyy');
      | else
      |     last = last(end-3:end);
      | end
      | 
      | if strcmp(first,last)
      |     fprintf('%s\nCopyright  %s Nexteer',NxtrConf,first);
      | else
      |     fprintf('%s\n%s%s-%s Nexteer',NxtrConf,char(169),first,last);
      | end
  Data Store Write : DataStoreWrite  DataStoreName=MotAg1CoeffTbl
  MotAg1CoeffTbl_SetRamBlockStatus : Subsystem
  wires:
  Block Changed = True/1 -> MotAg1CoeffTbl_SetRamBlockStatus/1(BlockChanged)
  MotAgCoeffTbl_ArgIn/1 -> Data Store Write/1

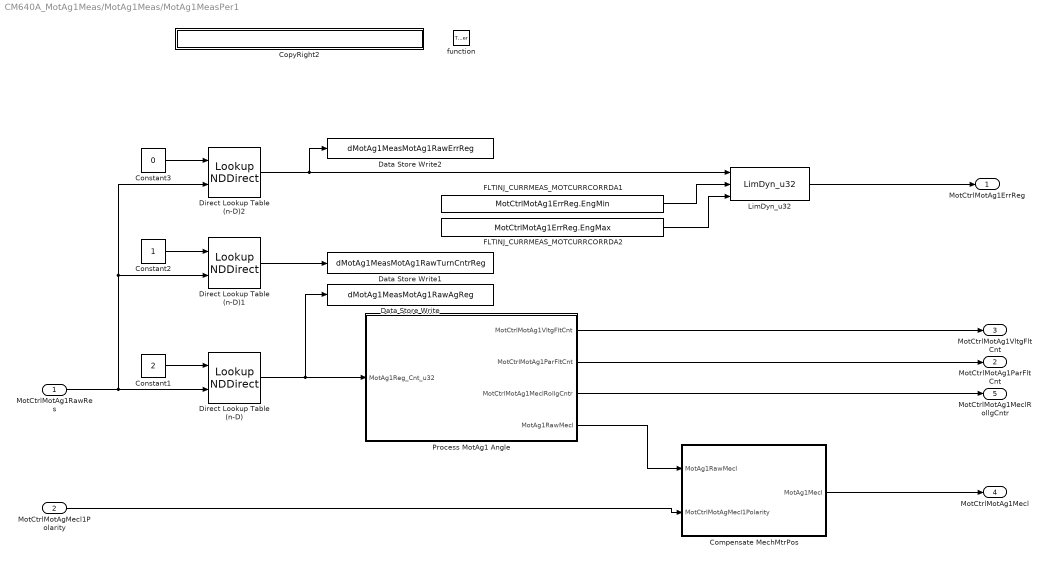
== system CM640A_MotAg1Meas/MotAg1Meas/MotAg1MeasPer1 ==
  MotCtrlMotAg1RawRes : Inport
  MotCtrlMotAgMecl1Polarity : Inport  Port=2
  function : TriggerPort  TriggerType=function-call
  Compensate MechMtrPos : Subsystem  RequirementInfo="{'linktype_rmi_doors' '0000cf48 (/ESG Group/FDD Module Requirements/EA4 Specific/CM640A_MotAg1Meas)' '#CM640A_95' 'true' 'REQ:  CM640A_95' '' ; 'linktype_rmi_doors' '0000cf48 (/ESG Group/FDD Module Requirements/EA4 Specific/CM640A_MotAg1Meas)' '#CM640A_89' 'true' 'REQ:  CM640A_89' '' } %GIDa_b988ae79_2e15_4ca3_aff9_cc168eec5403"
  Constant1 : Constant  Value=2
  Constant2 : Constant
  Constant3 : Constant  Value=0
  CopyRight2 : Subsystem  Description=|  mask(Copyright Information){none=on}
      | Copyright info block.                                               
      |                                                                     
      | Place copyright information at the top of every subsystem in design.
      mask prompts: none "No parameters"
      mask help: Place copyright information at the top of every subsystem in design.
      mask Display:
      | NxtrConf = 'Nexteer Confidential';
      | 
      | sys = bdroot; %handle for the current model ("system")
      | first = get_param(sys,'Created');
      | first = first(end-3:end);  %year is last four digits
      | 
      | last = get_param(sys,'LastModifiedDate');
      | if isempty(last)
      |     last = datestr(now,'yyyy');
      | else
      |     last = last(end-3:end);
      | end
      | 
      | if strcmp(first,last)
      |     fprintf('%s -- Copyright %s Nexteer',NxtrConf,first)
      | else
      |     fprintf('%s -- %s%s- %s Nexteer',NxtrConf,char(169),first,last)
      | end
  Data Store Write : DataStoreWrite  DataStoreName=dMotAg1MeasMotAg1RawAgReg
  Data Store Write1 : DataStoreWrite  DataStoreName=dMotAg1MeasMotAg1RawTurnCntrReg
  Data Store Write2 : DataStoreWrite  DataStoreName=dMotAg1MeasMotAg1RawErrReg
  Direct Lookup Table (n-D) : LookupNDDirect  NumberOfTableDimensions=1  TableIsInput=on
  Direct Lookup Table (n-D)1 : LookupNDDirect  NumberOfTableDimensions=1  TableIsInput=on
  Direct Lookup Table (n-D)2 : LookupNDDirect  NumberOfTableDimensions=1  TableIsInput=on
  FLTINJ_CURRMEAS_MOTCURRCORRDA1 : Constant  Value=MotCtrlMotAg1ErrReg.EngMin  OutDataTypeStr=uint32
  FLTINJ_CURRMEAS_MOTCURRCORRDA2 : Constant  Value=MotCtrlMotAg1ErrReg.EngMax  OutDataTypeStr=uint32
  LimDyn_u32 : NxtrLim/LimDyn_u32
  Process MotAg1 Angle : Subsystem  RequirementInfo="{'linktype_rmi_doors' '0000cf48 (/ESG Group/FDD Module Requirements/EA4 Specific/CM640A_MotAg1Meas)' '#CM640A_84' 'true' 'REQ:  CM640A_84' '' } %GIDa_44386883_ee1d_42a6_a5e7_3d37ab2a25a7"
  MotCtrlMotAg1ErrReg : Outport
  MotCtrlMotAg1ParFltCnt : Outport  Port=2
  MotCtrlMotAg1VltgFltCnt : Outport  Port=3
  MotCtrlMotAg1Mecl : Outport  Port=4
  MotCtrlMotAg1MeclRollgCntr : Outport  Port=5
  wires:
  Compensate MechMtrPos/1(MotAg1Mecl) -> MotCtrlMotAg1Mecl/1
  Constant1/1 -> Direct Lookup Table (n-D)/1
  MotCtrlMotAg1RawRes/1 -> Direct Lookup Table (n-D)2/2, Direct Lookup Table (n-D)1/2, Direct Lookup Table (n-D)/2
  Constant2/1 -> Direct Lookup Table (n-D)1/1
  Constant3/1 -> Direct Lookup Table (n-D)2/1
  Process MotAg1 Angle/1(MotCtrlMotAg1VltgFltCnt) -> MotCtrlMotAg1VltgFltCnt/1
  Process MotAg1 Angle/2(MotCtrlMotAg1ParFltCnt) -> MotCtrlMotAg1ParFltCnt/1
  MotCtrlMotAgMecl1Polarity/1 -> Compensate MechMtrPos/2(MotCtrlMotAgMecl1Polarity)
  Direct Lookup Table (n-D)2/1 -> LimDyn_u32/1, Data Store Write2/1
  Direct Lookup Table (n-D)1/1 -> Data Store Write1/1
  Direct Lookup Table (n-D)/1 -> Data Store Write/1, Process MotAg1 Angle/1(MotAg1Reg_Cnt_u32)
  Process MotAg1 Angle/3(MotCtrlMotAg1MeclRollgCntr) -> MotCtrlMotAg1MeclRollgCntr/1
  Process MotAg1 Angle/4(MotAg1RawMecl) -> Compensate MechMtrPos/1(MotAg1RawMecl)
  FLTINJ_CURRMEAS_MOTCURRCORRDA1/1 -> LimDyn_u32/2
  FLTINJ_CURRMEAS_MOTCURRCORRDA2/1 -> LimDyn_u32/3
  LimDyn_u32/1 -> MotCtrlMotAg1ErrReg/1

== system CM640A_MotAg1Meas/MotAg1Meas/MotAg1MeasPer2 ==
  MotAg1ErrReg : Inport
  MotAg1ParFltCnt : Inport  Port=2
  MotAg1VltgFltCnt : Inport  Port=3
  function : TriggerPort  TriggerType=function-call
  CopyRight2 : Subsystem  Description=|  mask(Copyright Information){none=on}
      | Copyright info block.                                               
      |                                                                     
      | Place copyright information at the top of every subsystem in design.
      mask prompts: none "No parameters"
      mask help: Place copyright information at the top of every subsystem in design.
      mask Display:
      | NxtrConf = 'Nexteer Confidential';
      | 
      | sys = bdroot; %handle for the current model ("system")
      | first = get_param(sys,'Created');
      | first = first(end-3:end);  %year is last four digits
      | 
      | last = get_param(sys,'LastModifiedDate');
      | if isempty(last)
      |     last = datestr(now,'yyyy');
      | else
      |     last = last(end-3:end);
      | end
      | 
      | if strcmp(first,last)
      |     fprintf('%s -- Copyright %s Nexteer',NxtrConf,first)
      | else
      |     fprintf('%s -- %s%s- %s Nexteer',NxtrConf,char(169),first,last)
      | end
  MotAg1 Protocol Fault Operation : Subsystem  RequirementInfo="{'linktype_rmi_doors' '0000cf48 (/ESG Group/FDD Module Requirements/EA4 Specific/CM640A_MotAg1Meas)' '#CM640A_106' 'true' 'REQ:  CM640A_106' '' } %GIDa_7fd546fd_48e1_4d9b_848f_bb77aa877077"
  Process ErrorReg and DieRevCtr : Subsystem  RequirementInfo="{'linktype_rmi_doors' '0000cf48 (/ESG Group/FDD Module Requirements/EA4 Specific/CM640A_MotAg1Meas)' '#CM640A_93' 'true' 'REQ:  CM640A_93' '' } %GIDa_46b1c473_7460_4468_9db5_508346730a23"
  MotAg1Qlfr : Outport  RequirementInfo={} %GIDa_3fc77e2f_6462_49ba_96ea_6336984b6724
  wires:
  MotAg1ErrReg/1 -> Process ErrorReg and DieRevCtr/1(MotAg1ErrReg)
  Process ErrorReg and DieRevCtr/1(MotAg1Err) -> MotAg1 Protocol Fault Operation/1(MotAg1Err)
  Process ErrorReg and DieRevCtr/2(MotAg1ErrParFltCnt) -> MotAg1 Protocol Fault Operation/2(MotAg1ErrParFltCnt)
  MotAg1 Protocol Fault Operation/1(MotAg1Qlfr) -> MotAg1Qlfr/1
  MotAg1ParFltCnt/1 -> MotAg1 Protocol Fault Operation/3(MotAg1ParFltCnt)
  MotAg1VltgFltCnt/1 -> MotAg1 Protocol Fault Operation/4(MotAg1VltgFltCnt)

== system CM640A_MotAg1Meas/Signal Creation/CopyRight2 ==

== system CM640A_MotAg1Meas/MotAg1Meas/MotAg1MeasInit1/Compute Correction Table ==
  CopyRight2 : Subsystem  Description=|  mask(Copyright Information){none=on}
      | Copyright info block.                                               
      |                                                                     
      | Place copyright information at the top of every subsystem in design.
      mask prompts: none "No parameters"
      mask help: Place copyright information at the top of every subsystem in design.
      mask Display:
      | NxtrConf = 'Nexteer Confidential';
      | 
      | sys = bdroot; %handle for the current model ("system")
      | first = get_param(sys,'Created');
      | first = first(end-3:end);  %year is last four digits
      | 
      | last = get_param(sys,'LastModifiedDate');
      | if isempty(last)
      |     last = datestr(now,'yyyy');
      | else
      |     last = last(end-3:end);
      | end
      | 
      | if strcmp(first,last)
      |     fprintf('%s -- Copyright %s Nexteer',NxtrConf,first)
      | else
      |     fprintf('%s -- %s%s- %s Nexteer',NxtrConf,char(169),first,last)
      | end
  If : If  IfExpression=u1 == 0
  MotAg1CorrnTbl_GetErrorStatus : Subsystem  TreatAsAtomicUnit=on
  NVM NOK : Subsystem  TreatAsAtomicUnit=on
  NVM Ok : Subsystem  TreatAsAtomicUnit=on
  wires:
  MotAg1CorrnTbl_GetErrorStatus/1(RequestResultPtr) -> If/1
  If/1 -> NVM Ok/Action
  If/2 -> NVM NOK/Action

== system CM640A_MotAg1Meas/MotAg1Meas/MotAg1MeasInit1/CopyRight2 ==

== system CM640A_MotAg1Meas/MotAg1Meas/MotAg1MeasInit1/Initialize CSIH RAM1 ==
  note: 1.  Configure the CSIH3 registers according to CM640A_MotAg1Meas_RegisterConfiguration.xlsm
      |     Order by Row.
  CopyRight2 : Subsystem  Description=|  mask(Copyright Information){none=on}
      | Copyright info block.                                               
      |                                                                     
      | Place copyright information at the top of every subsystem in design.
      mask prompts: none "No parameters"
      mask help: Place copyright information at the top of every subsystem in design.
      mask Display:
      | NxtrConf = 'Nexteer Confidential';
      | 
      | sys = bdroot; %handle for the current model ("system")
      | first = get_param(sys,'Created');
      | first = first(end-3:end);  %year is last four digits
      | 
      | last = get_param(sys,'LastModifiedDate');
      | if isempty(last)
      |     last = datestr(now,'yyyy');
      | else
      |     last = last(end-3:end);
      | end
      | 
      | if strcmp(first,last)
      |     fprintf('%s -- Copyright %s Nexteer',NxtrConf,first)
      | else
      |     fprintf('%s -- %s%s- %s Nexteer',NxtrConf,char(169),first,last)
      | end

== system CM640A_MotAg1Meas/MotAg1Meas/MotAg1MeasMotAg1CoeffTblRead/Copyright1 ==

== system CM640A_MotAg1Meas/MotAg1Meas/MotAg1MeasMotAg1CoeffTblWr/Copyright1 ==

== system CM640A_MotAg1Meas/MotAg1Meas/MotAg1MeasMotAg1CoeffTblWr/MotAg1CoeffTbl_SetRamBlockStatus ==
  note: This is the block representing the client call
  BlockChanged : Inport
  Terminator : Terminator
  wires:
  BlockChanged/1 -> Terminator/1

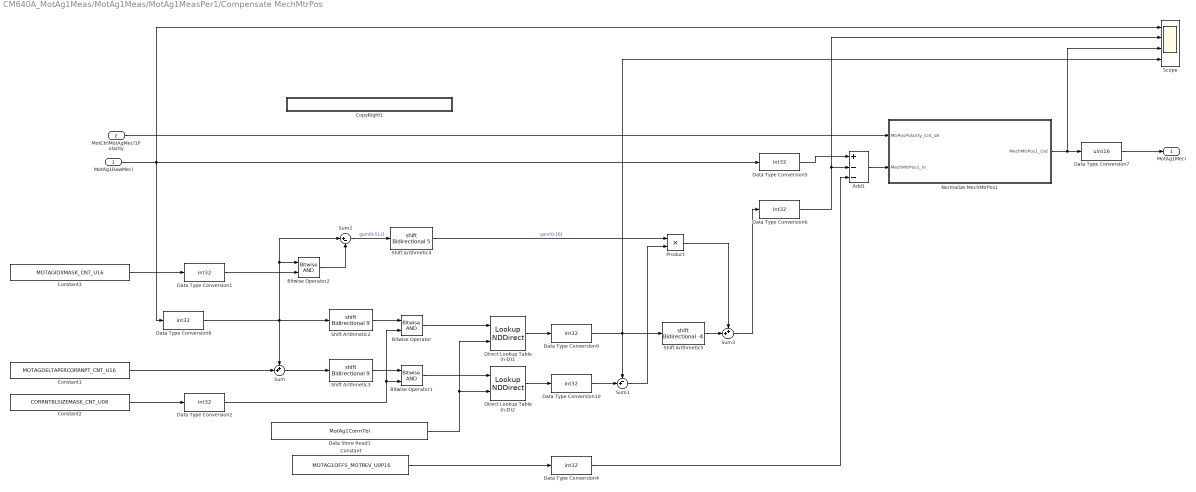
== system CM640A_MotAg1Meas/MotAg1Meas/MotAg1MeasPer1/Compensate MechMtrPos ==
  MotAg1RawMecl : Inport
  MotCtrlMotAgMecl1Polarity : Inport  Port=2
  Add1 : Sum  RequirementInfo="{'linktype_rmi_doors' '0000cf48 (/ESG Group/FDD Module Requirements/EA4 Specific/CM640A_MotAg1Meas)' '#CM640A_120' 'true' 'REQ:  CM640A_120' '' } %GIDa_6042ae8e_188c_4e3c_a559_115b77db5da1"  Inputs=+--
  Bitwise Operator : simulink/Logic and Bit Operations/Bitwise Operator  logicop=AND  UseBitMask=off  NumInputPorts=2  BitMask=CORRNTBLSIZEMASK_CNT_U08  BitMaskRealWorld=Stored Integer
  Bitwise Operator1 : simulink/Logic and Bit Operations/Bitwise Operator  logicop=AND  UseBitMask=off  NumInputPorts=2  BitMask=CORRNTBLSIZEMASK_CNT_U08  BitMaskRealWorld=Stored Integer
  Bitwise Operator2 : simulink/Logic and Bit Operations/Bitwise Operator  logicop=AND  UseBitMask=off  NumInputPorts=2  BitMask=MOTAGIDXMASK_CNT_U16  BitMaskRealWorld=Stored Integer
  Constant : Constant  Value=MOTAG1OFFS_MOTREV_U0P16
  Constant1 : Constant  Value=MOTAGDELTAPERCORRNPT_CNT_U16
  Constant2 : Constant  Value=CORRNTBLSIZEMASK_CNT_U08
  Constant3 : Constant  Value=MOTAGIDXMASK_CNT_U16
  CopyRight1 : Subsystem  Description=|  mask(Copyright Information){none=on}
      | Copyright info block.                                               
      |                                                                     
      | Place copyright information at the top of every subsystem in design.
      mask prompts: none "No parameters"
      mask help: Place copyright information at the top of every subsystem in design.
      mask Display:
      | NxtrConf = 'Nexteer Confidential';
      | 
      | sys = bdroot; %handle for the current model ("system")
      | first = get_param(sys,'Created');
      | first = first(end-3:end);  %year is last four digits
      | 
      | last = get_param(sys,'LastModifiedDate');
      | if isempty(last)
      |     last = datestr(now,'yyyy');
      | else
      |     last = last(end-3:end);
      | end
      | 
      | if strcmp(first,last)
      |     fprintf('%s -- Copyright %s Nexteer',NxtrConf,first)
      | else
      |     fprintf('%s -- %s%s- %s Nexteer',NxtrConf,char(169),first,last)
      | end
  Data Store Read1 : DataStoreRead  DataStoreName=MotAg1CorrnTbl
  Data Type Conversion{1..2,4..6,8..10} (8 alike) : DataTypeConversion  OutDataTypeStr=int32
  Data Type Conversion7 : DataTypeConversion  OutDataTypeStr=uint16
  Direct Lookup Table (n-D)1 : LookupNDDirect  NumberOfTableDimensions=1  TableIsInput=on
  Direct Lookup Table (n-D)2 : LookupNDDirect  NumberOfTableDimensions=1  TableIsInput=on
  Normalize MechMtrPos1 : Stateflow chart  RequirementInfo="{'linktype_rmi_doors' '0000cf48 (/ESG Group/FDD Module Requirements/EA4 Specific/CM640A_MotAg1Meas)' '#CM640A_90' 'true' 'REQ:  CM640A_90' '' } %GIDa_ea5b4198_0fe5_401b_8e9c_8665e43aa3b8"  TreatAsAtomicUnit=on
  Product : Product
  Scope : Scope  NumInputPorts=4
      settings: YMin=-5~-5~-5~-5  YMax=5~5~5~5
  Shift Arithmetic2 : ArithShift  BitShiftNumber=9
  Shift Arithmetic3 : ArithShift  BitShiftNumber=9
  Shift Arithmetic4 : ArithShift  BitShiftNumber=5
  Shift Arithmetic5 : ArithShift  BitShiftNumber=-4
  Sum : Sum  Inputs=++|
  Sum1 : Sum  Inputs=-+|
  Sum2 : Sum  Inputs=|+-
  Sum3 : Sum  Inputs=++|
  MotAg1Mecl : Outport
  wires:
  Constant/1 -> Data Type Conversion4/1
  Normalize MechMtrPos1/1(MechMtrPos1_Out) -> Scope/3, Data Type Conversion7/1
  MotCtrlMotAgMecl1Polarity/1 -> Normalize MechMtrPos1/1(MtrPosPolarity_Cnt_s8)
  Add1/1 -> Normalize MechMtrPos1/2(MechMtrPos1_In)
  Shift Arithmetic2/1 -> Bitwise Operator/1
  Data Type Conversion5/1 -> Add1/1
  Data Type Conversion6/1 -> Scope/2, Add1/2
  MotAg1RawMecl/1 -> Scope/1, Data Type Conversion5/1, Data Type Conversion8/1
  Data Type Conversion8/1 -> Sum/1, Sum2/1, Bitwise Operator2/1, Shift Arithmetic2/1
  Constant1/1 -> Sum/2
  Sum/1 -> Shift Arithmetic3/1
  Bitwise Operator/1 -> Direct Lookup Table (n-D)1/1
  Shift Arithmetic3/1 -> Bitwise Operator1/1
  Bitwise Operator1/1 -> Direct Lookup Table (n-D)2/1
  Data Store Read1/1 -> Direct Lookup Table (n-D)1/2, Direct Lookup Table (n-D)2/2
  Direct Lookup Table (n-D)1/1 -> Data Type Conversion9/1
  Direct Lookup Table (n-D)2/1 -> Data Type Conversion10/1
  Data Type Conversion9/1 -> Scope/4, Shift Arithmetic5/1, Sum1/1
  Data Type Conversion10/1 -> Sum1/2
  Bitwise Operator2/1 -> Sum2/2
  Sum2/1 -> Shift Arithmetic4/1  "gain(0-512)"
  Shift Arithmetic4/1 -> Product/1  "gain(0-16)"
  Sum1/1 -> Product/2
  Product/1 -> Sum3/1
  Shift Arithmetic5/1 -> Sum3/2
  Sum3/1 -> Data Type Conversion6/1
  Data Type Conversion4/1 -> Add1/3
  Data Type Conversion7/1 -> MotAg1Mecl/1
  Constant2/1 -> Data Type Conversion2/1
  Constant3/1 -> Data Type Conversion1/1
  Data Type Conversion1/1 -> Bitwise Operator2/2
  Data Type Conversion2/1 -> Bitwise Operator1/2, Bitwise Operator/2

== system CM640A_MotAg1Meas/MotAg1Meas/MotAg1MeasPer1/CopyRight2 ==

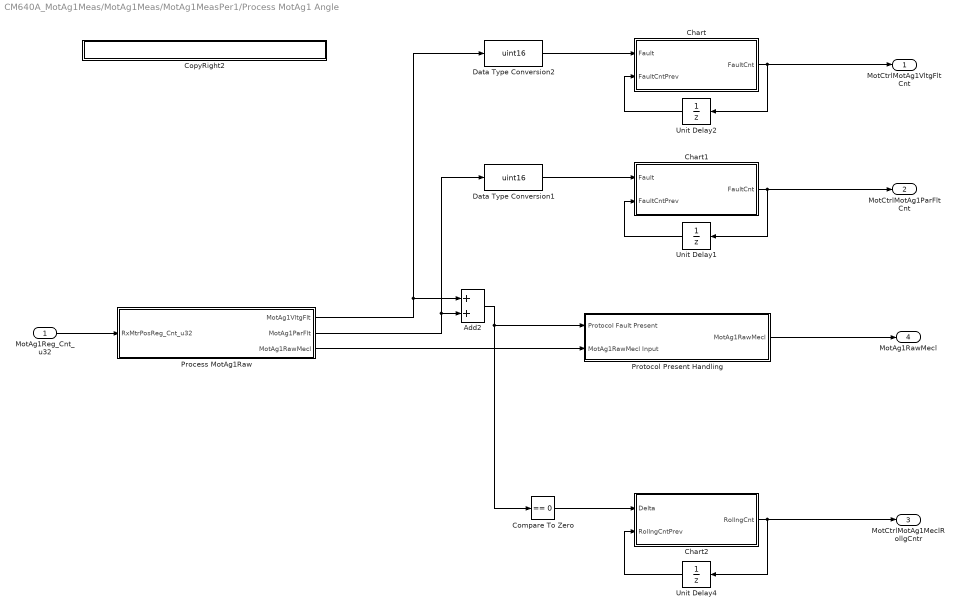
== system CM640A_MotAg1Meas/MotAg1Meas/MotAg1MeasPer1/Process MotAg1 Angle ==
  MotAg1Reg_Cnt_u32 : Inport
  Add2 : Sum  RequirementInfo="{'linktype_rmi_doors' '0000cf48 (/ESG Group/FDD Module Requirements/EA4 Specific/CM640A_MotAg1Meas)' '#CM640A_87' 'true' 'REQ:  CM640A_87' '' } %GIDa_0b7de0f8_fdb6_403a_993a_161f92b64634"
  Chart : Stateflow chart  TreatAsAtomicUnit=on
  Chart1 : Stateflow chart  TreatAsAtomicUnit=on
  Chart2 : Stateflow chart  RequirementInfo="{'linktype_rmi_doors' '0000cf48 (/ESG Group/FDD Module Requirements/EA4 Specific/CM640A_MotAg1Meas)' '#CM640A_107' 'true' 'REQ:  CM640A_107' '' } %GIDa_4e204d7d_fe00_4721_af4a_71a94d72e207"  TreatAsAtomicUnit=on
  Compare To Zero : simulink/Logic and Bit Operations/Compare To Zero  relop===  OutDataTypeStr=uint8
  CopyRight2 : Subsystem  Description=|  mask(Copyright Information){none=on}
      | Copyright info block.                                               
      |                                                                     
      | Place copyright information at the top of every subsystem in design.
      mask prompts: none "No parameters"
      mask help: Place copyright information at the top of every subsystem in design.
      mask Display:
      | NxtrConf = 'Nexteer Confidential';
      | 
      | sys = bdroot; %handle for the current model ("system")
      | first = get_param(sys,'Created');
      | first = first(end-3:end);  %year is last four digits
      | 
      | last = get_param(sys,'LastModifiedDate');
      | if isempty(last)
      |     last = datestr(now,'yyyy');
      | else
      |     last = last(end-3:end);
      | end
      | 
      | if strcmp(first,last)
      |     fprintf('%s -- Copyright %s Nexteer',NxtrConf,first)
      | else
      |     fprintf('%s -- %s%s- %s Nexteer',NxtrConf,char(169),first,last)
      | end
  Data Type Conversion1 : DataTypeConversion  OutDataTypeStr=uint16
  Data Type Conversion2 : DataTypeConversion  OutDataTypeStr=uint16
  Process MotAg1Raw : Subsystem  RequirementInfo={} %GIDa_f2e2859c_06d0_4da9_b7a1_6837a8f50074
  Protocol Present Handling : Subsystem  RequirementInfo="{'linktype_rmi_doors' '0000cf48 (/ESG Group/FDD Module Requirements/EA4 Specific/CM640A_MotAg1Meas)' '#CM640A_88' 'true' 'REQ:  CM640A_88' '' } %GIDa_d355b544_716b_4849_b17f_ed05c96132fe"  TreatAsAtomicUnit=on
  Unit Delay1 : UnitDelay  SampleTime=-1  StateName=MotAg1ParFltCntPrev  StateMustResolveToSignalObject=on
      settings: AttributesFormatString=|
      | State Variable:
      | %<StateName>
  Unit Delay2 : UnitDelay  SampleTime=-1  StateName=MotAg1VltgFltCntPrev  StateMustResolveToSignalObject=on
      settings: AttributesFormatString=|
      | State Variable:
      | %<StateName>
  Unit Delay4 : UnitDelay  SampleTime=-1  StateName=MotAg1MeclRollgCntrPrev  StateMustResolveToSignalObject=on
      settings: AttributesFormatString=|
      | State Variable:
      | %<StateName>
  MotCtrlMotAg1VltgFltCnt : Outport
  MotCtrlMotAg1ParFltCnt : Outport  Port=2
  MotCtrlMotAg1MeclRollgCntr : Outport  Port=3
  MotAg1RawMecl : Outport  Port=4
  wires:
  Add2/1 -> Compare To Zero/1, Protocol Present Handling/1(Protocol Fault Present)
  Process MotAg1Raw/1(MotAg1VltgFlt) -> Data Type Conversion2/1, Add2/1
  MotAg1Reg_Cnt_u32/1 -> Process MotAg1Raw/1(RxMtrPosReg_Cnt_u32)
  Process MotAg1Raw/2(MotAg1ParFlt) -> Data Type Conversion1/1, Add2/2
  Data Type Conversion2/1 -> Chart/1(Fault)
  Chart/1(FaultCnt) -> MotCtrlMotAg1VltgFltCnt/1, Unit Delay2/1
  Unit Delay2/1 -> Chart/2(FaultCntPrev)
  Data Type Conversion1/1 -> Chart1/1(Fault)
  Chart1/1(FaultCnt) -> MotCtrlMotAg1ParFltCnt/1, Unit Delay1/1
  Unit Delay1/1 -> Chart1/2(FaultCntPrev)
  Compare To Zero/1 -> Chart2/1(Delta)
  Chart2/1(RollngCnt) -> MotCtrlMotAg1MeclRollgCntr/1, Unit Delay4/1
  Unit Delay4/1 -> Chart2/2(RollngCntPrev)
  Process MotAg1Raw/3(MotAg1RawMecl) -> Protocol Present Handling/2(MotAg1RawMecl Input)
  Protocol Present Handling/1(MotAg1RawMecl) -> MotAg1RawMecl/1

== system CM640A_MotAg1Meas/MotAg1Meas/MotAg1MeasPer2/CopyRight2 ==

== system CM640A_MotAg1Meas/MotAg1Meas/MotAg1MeasPer2/MotAg1 Protocol Fault Operation ==
  note: Function Call Sequence Requirements
      |
      | - GetNtcQlfr shall execute after SetNtcSts
  MotAg1Err : Inport
  MotAg1ErrParFltCnt : Inport  Port=2
  MotAg1ParFltCnt : Inport  Port=3
  MotAg1VltgFltCnt : Inport  Port=4
  Atomic Subsystem : Subsystem  TreatAsAtomicUnit=on
  Constant : Constant  Value=MotAg1PrtclFlt
  CopyRight2 : Subsystem  Description=|  mask(Copyright Information){none=on}
      | Copyright info block.                                               
      |                                                                     
      | Place copyright information at the top of every subsystem in design.
      mask prompts: none "No parameters"
      mask help: Place copyright information at the top of every subsystem in design.
      mask Display:
      | NxtrConf = 'Nexteer Confidential';
      | 
      | sys = bdroot; %handle for the current model ("system")
      | first = get_param(sys,'Created');
      | first = first(end-3:end);  %year is last four digits
      | 
      | last = get_param(sys,'LastModifiedDate');
      | if isempty(last)
      |     last = datestr(now,'yyyy');
      | else
      |     last = last(end-3:end);
      | end
      | 
      | if strcmp(first,last)
      |     fprintf('%s -- Copyright %s Nexteer',NxtrConf,first)
      | else
      |     fprintf('%s -- %s%s- %s Nexteer',NxtrConf,char(169),first,last)
      | end
  Data store for model purposes only - don't code : DataStoreMemory  DataStoreName=NtcQlfr  ReadBeforeWriteMsg=warning  WriteAfterWriteMsg=warning  WriteAfterReadMsg=warning
  GetNtcQlfr : Subsystem  RequirementInfo={} %GIDa_2788174b_a957_4dc9_a642_eff6dc86ed2e
  Scope : Scope  NumInputPorts=3
      settings: YMin=-5~-5~-5  YMax=5~5~5  SaveName=ScopeData4
  SetNtcSts : Subsystem  RequirementInfo="{'linktype_rmi_doors' '0000cf48 (/ESG Group/FDD Module Requirements/EA4 Specific/CM640A_MotAg1Meas)' '#CM640A_22' 'true' 'REQ:  CM640A_22' '' } %GIDa_20dd2f86_c7d6_4283_b0b0_3f19883521de"
  Subsystem : Subsystem  RequirementInfo="{'linktype_rmi_doors' '0000cf48 (/ESG Group/FDD Module Requirements/EA4 Specific/CM640A_MotAg1Meas)' '#CM640A_111' 'true' 'REQ:  CM640A_111' '' ; 'linktype_rmi_doors' '0000cf48 (/ESG Group/FDD Module Requirements/EA4 Specific/CM640A_MotAg1Meas)' '#CM640A_25' 'true' 'REQ:  CM640A_25' '' } %GIDa_b90c0a5c_15cf_4b9e_8505_312514bbc1da"
  MotAg1Qlfr : Outport  RequirementInfo={} %GIDa_cf1cbe4f_1681_476d_80fb_f928627be900
  wires:
  MotAg1Err/1 -> Subsystem/1(MotAg1Err)
  MotAg1ErrParFltCnt/1 -> Subsystem/2(MotAg1ErrParFltCnt)
  MotAg1ParFltCnt/1 -> Subsystem/3(MotAg1ParFltCnt)
  MotAg1VltgFltCnt/1 -> Subsystem/4(MotAg1VltgFltCnt)
  Constant/1 -> GetNtcQlfr/1(NtcNr), SetNtcSts/1(NtcNr)  "NtcNr"
  Subsystem/1(NtcStInfo) -> Scope/1, Atomic Subsystem/1(NtcStInfo), SetNtcSts/2(NtcStInfo)  "ParamByte"
  GetNtcQlfr/1(NtcQlfr) -> Scope/3, MotAg1Qlfr/1
  Atomic Subsystem/1(NtcSts) -> SetNtcSts/3(NtcSts)
  Atomic Subsystem/2(DebStep) -> SetNtcSts/4(DebStep), Scope/2
